simulink model "oloop1"  (Simulink 10.0)
settings: Solver=ode15s  StartTime=0.0  StopTime=120  MaxStep=1  RelTol=1e-3  AbsTol=1e-3
undefined symbols (not defined in the file): sfunyst, uaero0, uprop0
libraries: simulink3 x6, fbuttons x5, fdctools x3, fdclib10 x1
settings Model: Creator=bhisma  LastModifiedBy=bhisma  ExtModeTrigMode=oneshot  ExtModeArmWhenConnect=off
settings DataIOCC: SignalLoggingSaveFormat=ModelDataLogs  SaveOutput=off  SaveTime=off  Refine=4
settings OptimizationCC: BlockReduction=off  BooleanDataType=off  LifeSpan=auto
settings DebuggingCC: SaveWithParameterizedLinksMsg=none  SignalResolutionControl=TryResolveAllWithWarning  MultiTaskDSMMsg=warning  MultiTaskCondExecSysMsg=none  SFUnexpectedBacktrackingDiag=error  SFNoUnconditionalDefaultTransitionDiag=error  SFExecutionAtInitializationDiag=warning  ArithmeticOperatorsInVariantConditions=error
settings HardwareCC: ProdBitPerPointer=64  ProdBitPerSizeT=64  ProdBitPerPtrDiffT=64  ProdLargestAtomicFloat=Float  ProdIntDivRoundTo=Zero  ProdEndianess=LittleEndian  ProdWordSize=64  ProdHWDeviceType=Intel->x86-64 (Windows64)  TargetUnknown=on
settings SFSimCC: SimUseLocalCustomCode=on  CustomCodeUndefinedFunction=FilterOut
settings RTWCC: TemplateMakefile=grt_vc.tmf  RTWUseLocalCustomCode=on
settings CodeAppCC: StateflowObjectComments=off
settings GRTTargetCC: TargetLangStandard=C99 (ISO)
settings ConfigComp: CovMetricSettings=dwe  CovHtmlReporting=off  CovSaveCumulativeToWorkspaceVar=off  CovSaveSingleToWorkspaceVar=off

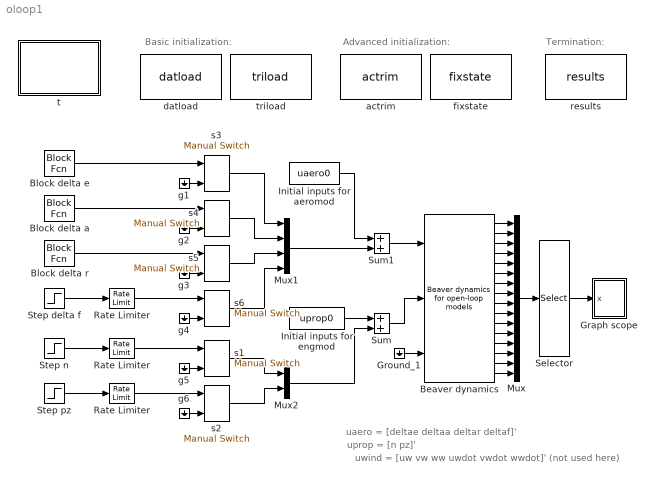
== system oloop1 ==
  note: Basic initialization:
  note: uaero = [deltae deltaa deltar deltaf]'
  note: uprop = [n pz]'
  note: uwind = [uw vw ww uwdot vwdot wwdot]' (not used here)
  note: Termination:
  note: Advanced initialization:
  " Rate Limiter" : RateLimiter  RisingSlewLimit=1.0  FallingSlewLimit=-1.0
  Beaver dynamics : fdclib10/Beaver dynamics  for open-loop models
  Block delta a : fdctools/Block Fcn  yinit=0  yblock=3*pi/180  tstart=0.001  tstop=2
  Block delta e : fdctools/Block Fcn  yinit=0  yblock=3*pi/180  tstart=0.001  tstop=2
  Block delta r : fdctools/Block Fcn  yinit=0  yblock=3*pi/180  tstart=0.001  tstop=2
  Graph scope : Subsystem  mask(Storage scope.){Parameter1=10, Parameter2=-10, Parameter3=10, npts=100, color='g-'}
      mask prompts: Parameter1 "Initial Time Range:"; Parameter2 "Initial y-min:"; Parameter3 "Initial y-max:"; npts "Storage pts.:"; color "Line type (rgbw-.:xo):"
      mask help:
      | Storage scope using MATLAB graph window.
      | Enter plotting ranges and line type.
      mask init:
      | close all; ax = [0, @1, @2, @3];
      mask Help: Uses MATLAB's graph window.\nUse only one block per system.\nLine type must be in quotes.\nSee the M-file sfunyst.m.
      mask Display: plot(0,0,100,100,[83,76,63,52,42,38,28,16,11,84,11,11,11,90,90,11],[75,58,47,54,72,80,84,74,65,65,65,90,40,40,90,90])
  Ground_1 : Ground
  Initial inputs for aeromod : Constant  Value=uaero0
  Initial inputs for engmod : Constant  Value=uprop0
  Mux : Mux  Inputs=16
  Mux1 : Mux
  Mux2 : Mux  Inputs=2
  Rate Limiter : RateLimiter  RisingSlewLimit=pi/180  FallingSlewLimit=-pi/180
  "Rate Limiter " : RateLimiter  RisingSlewLimit=50  FallingSlewLimit=-50
  Selector : Selector  InputPortWidth=16  IndexOptions=Index vector (dialog)  Indices=8  OutputSizes=1
  Step delta f : Step  Time=0.001  After=3*pi/180  SampleTime=0
  Step n : Step  Time=0.001  After=200  SampleTime=0
  Step pz : Step  Time=0.001  After=2  SampleTime=0
  Sum : Sum  SaturateOnIntegerOverflow=on  InputSameDT=on  OutDataTypeStr=Inherit: Same as first input
  Sum1 : Sum  SaturateOnIntegerOverflow=on  InputSameDT=on  OutDataTypeStr=Inherit: Same as first input
  actrim : fbuttons/actrim
  datload : fbuttons/datload
  fixstate : fbuttons/fixstate
  g{1..6} (6 alike) : Ground
  results : fbuttons/results
  s{1..2,4..6} (5 alike) : simulink3/Nonlinear/Manual Switch  sw=0  action=0
      settings: SourceProductName=Simulink  SourceProductBaseCode=SL
  s3 : simulink3/Nonlinear/Manual Switch  sw=1  action=0
      settings: SourceProductName=Simulink  SourceProductBaseCode=SL
  t : Subsystem
      settings: OpenFcn=browse oloop
      mask Display: disp('OLOOP1\nMarc Rauw\nJanuary 2004')
  triload : fbuttons/triload
  wires:
  Step delta f/1 -> Rate Limiter/1
  Ground_1/1 -> Beaver dynamics/3
  Sum1/1 -> Beaver dynamics/1
  Initial inputs for engmod/1 -> Sum/1
  Sum/1 -> Beaver dynamics/2
  g5/1 -> s1/2
  g6/1 -> s2/2
  Initial inputs for aeromod/1 -> Sum1/1
  Mux1/1 -> Sum1/2
  g1/1 -> s3/2
  g4/1 -> s6/2
  g3/1 -> s5/2
  g2/1 -> s4/2
  s6/1 -> Mux1/4
  s5/1 -> Mux1/3
  s4/1 -> Mux1/2
  s3/1 -> Mux1/1
  Mux2/1 -> Sum/2
  Rate Limiter/1 -> s6/1
  s2/1 -> Mux2/2
  s1/1 -> Mux2/1
  "Rate Limiter "/1 -> s1/1
  Step n/1 -> "Rate Limiter "/1
  Step pz/1 -> " Rate Limiter"/1
  " Rate Limiter"/1 -> s2/1
  Block delta r/1 -> s5/1
  Block delta a/1 -> s4/1
  Block delta e/1 -> s3/1
  Selector/1 -> Graph scope/1(x)
  Beaver dynamics/1 -> Mux/1
  Beaver dynamics/2 -> Mux/2
  Beaver dynamics/3 -> Mux/3
  Beaver dynamics/4 -> Mux/4
  Beaver dynamics/5 -> Mux/5
  Beaver dynamics/6 -> Mux/6
  Beaver dynamics/7 -> Mux/7
  Beaver dynamics/8 -> Mux/8
  Beaver dynamics/9 -> Mux/9
  Beaver dynamics/10 -> Mux/10
  Beaver dynamics/11 -> Mux/11
  Beaver dynamics/12 -> Mux/12
  Beaver dynamics/13 -> Mux/13
  Beaver dynamics/14 -> Mux/14
  Beaver dynamics/15 -> Mux/15
  Beaver dynamics/16 -> Mux/16
  Mux/1 -> Selector/1

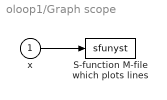
== system oloop1/Graph scope ==
  x : Inport
  "S-function M-file which plots lines " : S-Function  LoadFcn=sfunyst([],[],[],'LoadBlock')  FunctionName=sfunyst  Parameters=ax, color, npts  SFunctionDeploymentMode=off  EnableBusSupport=off
      settings: CopyFcn=sfunyst([],[],[],'CopyBlock')  DeleteFcn=sfunyst([],[],[],'DeleteBlock')
  wires:
  x/1 -> "S-function M-file which plots lines "/1

== system oloop1/t ==
